simulink model "controller_position_east"  (R2020a)
settings: Solver=FixedStepAuto  StartTime=0.0  StopTime=10.0  FixedStep=1/sim_freq  RelTol=1e-3
undefined symbols (not defined in the file): G_PE_OL_DENOM, G_PE_OL_NUM, K_ep
settings Model: Creator=francois  LastModifiedBy=murray

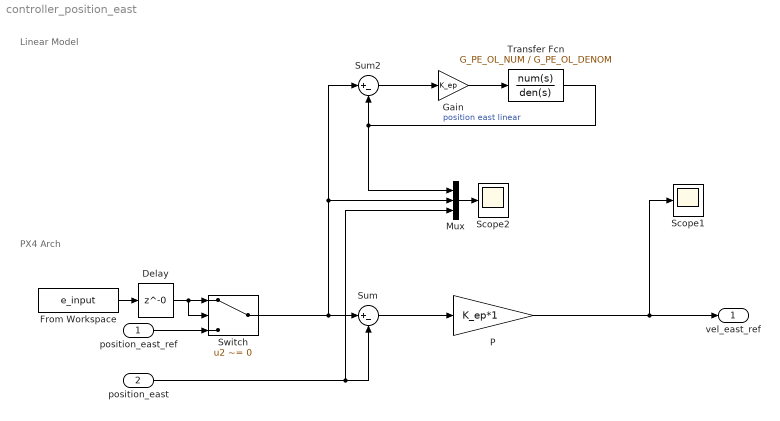
== system controller_position_east ==
  note: Linear Model
  note: PX4 Arch
  position_east_ref : Inport
  position_east : Inport  Port=2
  Delay : Delay  DelayLength=0
  From Workspace : FromWorkspace  VariableName=e_input
  Gain : Gain  Gain=K_ep
  Mux : Mux  Inputs=3
  P : Gain  Gain=K_ep*1
  Scope1 : Scope
  Scope2 : Scope
  Sum : Sum  Inputs=|+-
  Sum2 : Sum  Inputs=|+-
  Switch : Switch  Criteria=u2 ~= 0
  Transfer Fcn : TransferFcn  Numerator=G_PE_OL_NUM  Denominator=G_PE_OL_DENOM
  vel_east_ref : Outport  VectorParamsAs1DForOutWhenUnconnected=off
  wires:
  Switch/1 -> Sum/1, Mux/2, Sum2/1
  Sum2/1 -> Gain/1
  P/1 -> vel_east_ref/1, Scope1/1
  position_east/1 -> Mux/3, Sum/2
  From Workspace/1 -> Delay/1
  Gain/1 -> Transfer Fcn/1
  Transfer Fcn/1 -> Mux/1, Sum2/2  "position east linear"
  Sum/1 -> P/1
  Delay/1 -> Switch/2, Switch/1
  position_east_ref/1 -> Switch/3
  Mux/1 -> Scope2/1
